simulink model "pid_2dof_nonlinear_c_speed"  (R2017a)
settings: Solver=ode45  StartTime=0.0  StopTime=5  RelTol=1e-3
undefined symbols (not defined in the file): f, g, GoalPos, k_p, l, m_p
libraries: simulink x2
settings Model: Creator=sansh  LastModifiedBy=rj2318

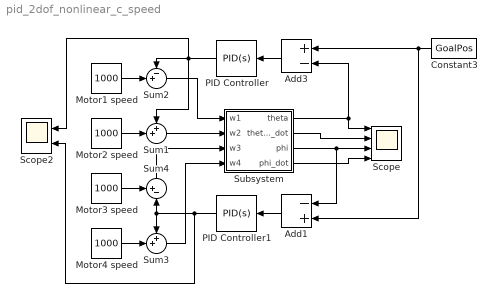
== system pid_2dof_nonlinear_c_speed ==
  Add1 : Sum  Inputs=-+
  Add3 : Sum  Inputs=+-
  Constant3 : Constant  Value=GoalPos
  Motor1 speed : Constant  Value=1000
  Motor2 speed : Constant  Value=1000
  Motor3 speed : Constant  Value=1000
  Motor4 speed : Constant  Value=1000
  PID Controller : simulink/Continuous/PID Controller  Controller=PID  TimeDomain=Continuous-time  SampleTime=-1  IntegratorMethod=Forward Euler  FilterMethod=Forward Euler  Form=Parallel  UseFilter=on  ControllerParametersSource=internal  P=100  I=0.1  D=100  N=10  InitialConditionSource=internal  InitialConditionForIntegrator=0  InitialConditionForFilter=0  ExternalReset=none  LimitOutput=off  UpperSaturationLimit=inf  LowerSaturationLimit=-inf  LinearizeAsGain=on  AntiWindupMode=none  Kb=1  TrackingMode=off  Kt=1  PParamMin=[]  PParamMax=[]  IParamMin=[]  IParamMax=[]  DParamMin=[]  DParamMax=[]  NParamMin=[]  NParamMax=[]  KbParamMin=[]  KbParamMax=[]  KtParamMin=[]  KtParamMax=[]  POutMin=[]  POutMax=[]  IOutMin=[]  IOutMax=[]  DOutMin=[]  DOutMax=[]  NOutMin=[]  NOutMax=[]  KbOutMin=[]  KbOutMax=[]  KtOutMin=[]  KtOutMax=[]  IntegratorOutMin=[]  IntegratorOutMax=[]  FilterOutMin=[]  FilterOutMax=[]  SumOutMin=[]  SumOutMax=[]  SumI1OutMin=[]  SumI1OutMax=[]  SumI2OutMin=[]  SumI2OutMax=[]  SumI3OutMin=[]  SumI3OutMax=[]  SumDOutMin=[]  SumDOutMax=[]  SaturationOutMin=[]  SaturationOutMax=[]  IntegratorContinuousStateAttributes=''  IntegratorStateMustResolveToSignalObject=off  IntegratorRTWStateStorageClass=Auto  FilterContinuousStateAttributes=''  FilterStateMustResolveToSignalObject=off  FilterRTWStateStorageClass=Auto  DifferentiatorICPrevScaledInput=0  DifferentiatorOutMin=[]  DifferentiatorOutMax=[]
  PID Controller1 : simulink/Continuous/PID Controller  Controller=PID  TimeDomain=Continuous-time  SampleTime=-1  IntegratorMethod=Forward Euler  FilterMethod=Forward Euler  Form=Parallel  UseFilter=on  ControllerParametersSource=internal  P=100  I=0.01  D=10  N=10  InitialConditionSource=internal  InitialConditionForIntegrator=0  InitialConditionForFilter=0  ExternalReset=none  LimitOutput=off  UpperSaturationLimit=inf  LowerSaturationLimit=-inf  LinearizeAsGain=on  AntiWindupMode=none  Kb=1  TrackingMode=off  Kt=1  PParamMin=[]  PParamMax=[]  IParamMin=[]  IParamMax=[]  DParamMin=[]  DParamMax=[]  NParamMin=[]  NParamMax=[]  KbParamMin=[]  KbParamMax=[]  KtParamMin=[]  KtParamMax=[]  POutMin=[]  POutMax=[]  IOutMin=[]  IOutMax=[]  DOutMin=[]  DOutMax=[]  NOutMin=[]  NOutMax=[]  KbOutMin=[]  KbOutMax=[]  KtOutMin=[]  KtOutMax=[]  IntegratorOutMin=[]  IntegratorOutMax=[]  FilterOutMin=[]  FilterOutMax=[]  SumOutMin=[]  SumOutMax=[]  SumI1OutMin=[]  SumI1OutMax=[]  SumI2OutMin=[]  SumI2OutMax=[]  SumI3OutMin=[]  SumI3OutMax=[]  SumDOutMin=[]  SumDOutMax=[]  SaturationOutMin=[]  SaturationOutMax=[]  IntegratorContinuousStateAttributes=''  IntegratorStateMustResolveToSignalObject=off  IntegratorRTWStateStorageClass=Auto  FilterContinuousStateAttributes=''  FilterStateMustResolveToSignalObject=off  FilterRTWStateStorageClass=Auto  DifferentiatorICPrevScaledInput=0  DifferentiatorOutMin=[]  DifferentiatorOutMax=[]
  Scope : Scope  NumInputPorts=4
  Scope2 : Scope  NumInputPorts=2
  Subsystem : Subsystem
  Sum1 : Sum  Inputs=++|
  Sum2 : Sum  Inputs=-+|
  Sum3 : Sum  Inputs=++|
  Sum4 : Sum  Inputs=+-|
  wires:
  Subsystem/1(theta) -> Add3/2, Scope/1
  Subsystem/2(theta_dot) -> Scope/2
  Add3/1 -> PID Controller/1
  Subsystem/3(phi) -> Add1/1, Scope/3
  Constant3/1 -> Add3/1, Add1/2
  Subsystem/4(phi_dot) -> Scope/4
  Add1/1 -> PID Controller1/1
  Sum3/1 -> Subsystem/4(w4)
  Motor3 speed/1 -> Sum4/1
  PID Controller1/1 -> Scope2/2, Sum4/2, Sum3/1
  Motor4 speed/1 -> Sum3/2
  PID Controller/1 -> Scope2/1, Sum2/1, Sum1/1
  Sum4/1 -> Subsystem/3(w3)
  Sum1/1 -> Subsystem/2(w2)
  Sum2/1 -> Subsystem/1(w1)
  Motor1 speed/1 -> Sum2/2
  Motor2 speed/1 -> Sum1/2

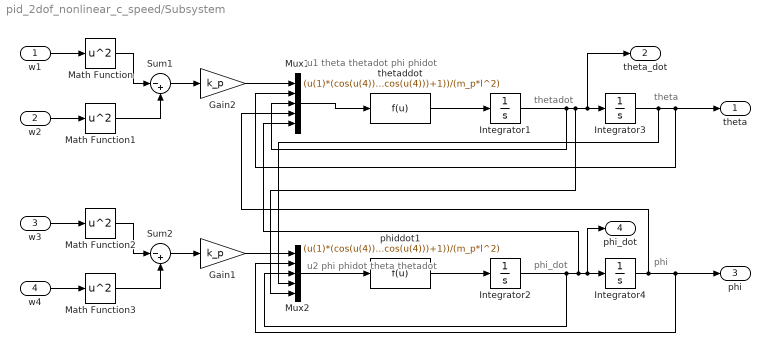
== system pid_2dof_nonlinear_c_speed/Subsystem ==
  note: theta
  note: thetadot
  note: phi
  note: phi_dot
  note: u1
      | theta
      | thetadot
      | phi
      | phidot
  note: u2
      | phi
      | phidot
      | theta
      | thetadot
  w1 : Inport
  w2 : Inport  Port=2
  w3 : Inport  Port=3
  w4 : Inport  Port=4
  Gain1 : Gain  Gain=k_p
  Gain2 : Gain  Gain=k_p
  Integrator1 : Integrator  ContinuousStateAttributes='thetadot'
  Integrator2 : Integrator  ContinuousStateAttributes='thetadot'
  Integrator3 : Integrator  InitialCondition=0.1  ContinuousStateAttributes='theta'
  Integrator4 : Integrator  InitialCondition=0.1  ContinuousStateAttributes='theta'
  Math Function{,1..3} (4 alike) : Math  Operator=square  SaturateOnIntegerOverflow=on
  Mux1 : Mux  Inputs=5
  Mux2 : Mux  Inputs=5
  Sum1 : Sum  Inputs=|-+
  Sum2 : Sum  Inputs=|-+
  phiddot1 : Fcn  Expr=(u(1)*(cos(u(4))+cos(u(2))*sin(u(4))^2)-(u(3)^2)*f*l^2+m_p*g*l*sin(u(2))*sqrt(((cos(u(2))*sin(u(4))^2)/cos(u(4)))+1))/(m_p*l^2)
  thetaddot : Fcn  Expr=(u(1)*(cos(u(4))+cos(u(2))*sin(u(4))^2)-(u(3)^2)*f*l^2+m_p*g*l*sin(u(2))*sqrt(((cos(u(2))*sin(u(4))^2)/cos(u(4)))+1))/(m_p*l^2)
  theta : Outport
  theta_dot : Outport  Port=2
  phi : Outport  Port=3
  phi_dot : Outport  Port=4
  wires:
  Mux1/1 -> thetaddot/1
  thetaddot/1 -> Integrator1/1
  Integrator1/1 -> Mux1/3, Mux2/5, theta_dot/1, Integrator3/1
  Integrator3/1 -> Mux2/4, Mux1/2, theta/1
  Integrator4/1 -> Mux2/2, phi/1, Mux1/4
  phiddot1/1 -> Integrator2/1
  Mux2/1 -> phiddot1/1
  Integrator2/1 -> Mux2/3, Mux1/5, phi_dot/1, Integrator4/1
  w3/1 -> Math Function2/1
  Math Function3/1 -> Sum2/2
  Math Function/1 -> Sum1/1
  w1/1 -> Math Function/1
  w4/1 -> Math Function3/1
  Math Function1/1 -> Sum1/2
  Sum1/1 -> Gain2/1
  Gain2/1 -> Mux1/1
  Sum2/1 -> Gain1/1
  w2/1 -> Math Function1/1
  Math Function2/1 -> Sum2/1
  Gain1/1 -> Mux2/1
